simulink model "system_FIR_bank_decoder_AWGN"  (Simulink 8.3)
settings: Solver=ode45  StartTime=0.0  StopTime=10  RelTol=1e-3
undefined symbols (not defined in the file or in its folder): fdesignblkfcn, gcbh
libraries: commutil2 x2, commchan3 x1
(part 1 of 2)
settings Model: Creator=Vasilis  LastModifiedBy=Vasilis
settings OptimizationCC: ExpressionDepthLimit=2147483647
settings DebuggingCC: FcnCallInpInsideContextMsg=UseLocalSettings

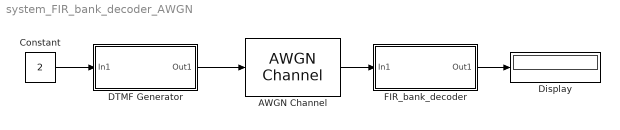
== system system_FIR_bank_decoder_AWGN ==
  AWGN Channel : commchan3/AWGN Channel  InputProcessing=Columns as channels (frame based)  seed=67  noiseMode="Signal to noise ratio  (SNR)"  EbNodB=10  EsNodB=10  SNRdB=-6  bitsPerSym=1  Ps=1  Tsym=1  variance=1
  Constant : Constant  Value=2
  DTMF Generator : Subsystem
  Display : Display
  FIR_bank_decoder : Subsystem
  wires:
  DTMF Generator/1(Out1) -> AWGN Channel/1
  FIR_bank_decoder/1(Out1) -> Display/1
  Constant/1 -> DTMF Generator/1(In1)
  AWGN Channel/1 -> FIR_bank_decoder/1(In1)

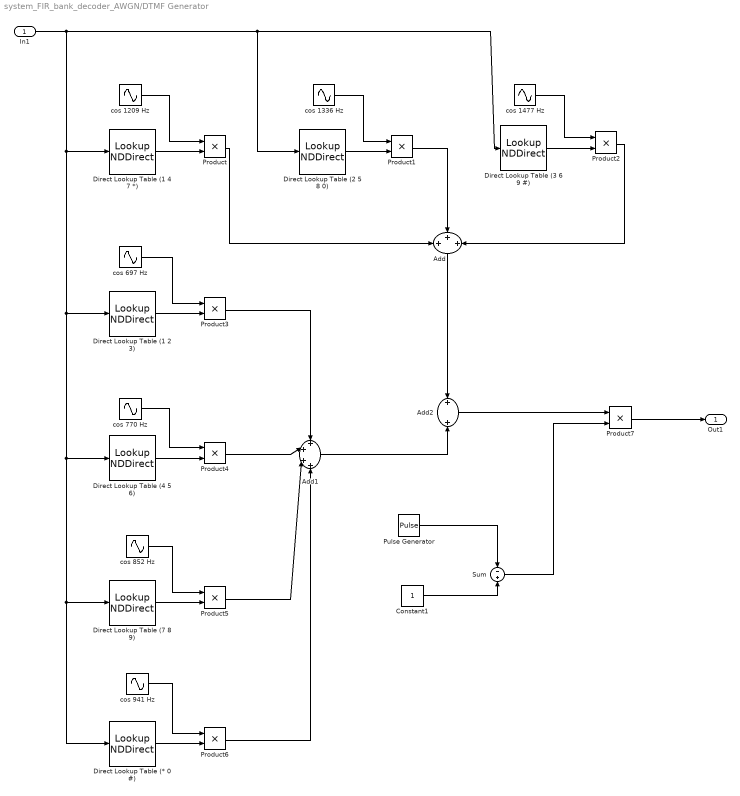
== system system_FIR_bank_decoder_AWGN/DTMF Generator ==
  In1 : Inport
  Add : Sum  Inputs=+++
  Add1 : Sum  Inputs=++++
  Add2 : Sum
  Constant1 : Constant
  Direct Lookup Table (* 0 #) : LookupNDDirect  NumberOfTableDimensions=1  Table=[1 0 0 0 0 0 0 0 0 0 1 1]
  Direct Lookup Table (1 2 3) : LookupNDDirect  NumberOfTableDimensions=1  Table=[0 1 1 1 0 0 0 0 0 0 0 0]
  Direct Lookup Table (1 4 7 *) : LookupNDDirect  NumberOfTableDimensions=1  Table=[0 1 0 0 1 0 0 1 0 0 1 0]
  Direct Lookup Table (2 5 8 0) : LookupNDDirect  NumberOfTableDimensions=1  Table=[1 0 1 0 0 1 0 0 1 0 0 0]
  Direct Lookup Table (3 6 9 #) : LookupNDDirect  NumberOfTableDimensions=1  Table=[0 0 0 1 0 0 1 0 0 1 0 1]
  Direct Lookup Table (4 5 6) : LookupNDDirect  NumberOfTableDimensions=1  Table=[0 0 0 0 1 1 1 0 0 0 0 0]
  Direct Lookup Table (7 8 9) : LookupNDDirect  NumberOfTableDimensions=1  Table=[0 0 0 0 0 0 0 1 1 1 0 0]
  Product{,1..7} (8 alike) : Product  RndMeth=Zero
  Pulse Generator : DiscretePulseGenerator  Period=480  PulseWidth=160  PhaseDelay=320  SampleTime=1/8000
  Sum : Sum  Inputs=-|+
  cos 1209 Hz : Sin  Frequency=7596  Phase=pi/2  SampleTime=1/8000
  cos 1336 Hz : Sin  Frequency=8394  Phase=pi/2  SampleTime=1/8000
  cos 1477 Hz : Sin  Frequency=9280  Phase=pi/2  SampleTime=1/8000
  cos 697 Hz : Sin  Frequency=4379  Phase=pi/2  SampleTime=1/8000
  cos 770 Hz : Sin  Frequency=4838  Phase=pi/2  SampleTime=1/8000
  cos 852 Hz : Sin  Frequency=5353  Phase=pi/2  SampleTime=1/8000
  cos 941 Hz : Sin  Frequency=5912  Phase=pi/2  SampleTime=1/8000
  Out1 : Outport
  wires:
  Direct Lookup Table (1 4 7 *)/1 -> Product/2
  In1/1 -> Direct Lookup Table (2 5 8 0)/1, Direct Lookup Table (3 6 9 #)/1, Direct Lookup Table (1 4 7 *)/1, Direct Lookup Table (1 2 3)/1, Direct Lookup Table (4 5 6)/1, Direct Lookup Table (7 8 9)/1, Direct Lookup Table (* 0 #)/1
  cos 1336 Hz/1 -> Product1/1
  Direct Lookup Table (2 5 8 0)/1 -> Product1/2
  cos 1477 Hz/1 -> Product2/1
  Direct Lookup Table (3 6 9 #)/1 -> Product2/2
  cos 697 Hz/1 -> Product3/1
  Direct Lookup Table (1 2 3)/1 -> Product3/2
  cos 770 Hz/1 -> Product4/1
  Direct Lookup Table (4 5 6)/1 -> Product4/2
  cos 852 Hz/1 -> Product5/1
  Direct Lookup Table (7 8 9)/1 -> Product5/2
  Product2/1 -> Add/3
  Product1/1 -> Add/2
  Product/1 -> Add/1
  Product3/1 -> Add1/1
  Product5/1 -> Add1/3
  Product4/1 -> Add1/2
  Add1/1 -> Add2/2
  Add/1 -> Add2/1
  cos 941 Hz/1 -> Product6/1
  Direct Lookup Table (* 0 #)/1 -> Product6/2
  Product6/1 -> Add1/4
  cos 1209 Hz/1 -> Product/1
  Constant1/1 -> Sum/2
  Pulse Generator/1 -> Sum/1
  Product7/1 -> Out1/1
  Add2/1 -> Product7/1
  Sum/1 -> Product7/2

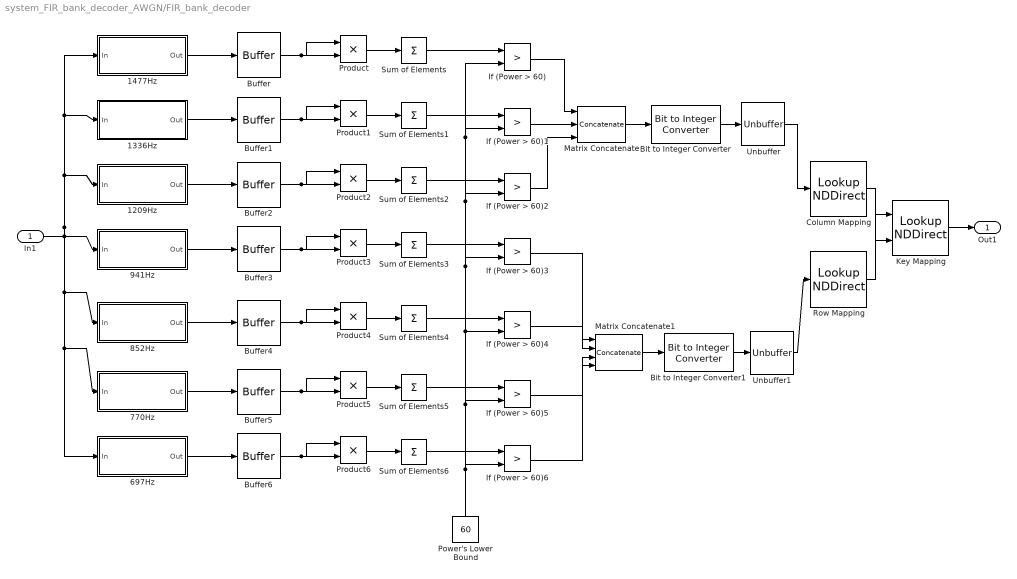
== system system_FIR_bank_decoder_AWGN/FIR_bank_decoder ==
  In1 : Inport
  1209Hz : Subsystem  DialogController=fdesignblkfcn  DialogControllerArgs=DataTag2  InitFcn=fdesignblkfcn(gcbh, {'InitFcn'});  mask(Bandpass Filter){}
      mask help: Design a bandpass filter
      settings: CopyFcn=fdesignblkfcn(gcbh, {'CopyFcn'});
      mask Help: helpview(mapfilelocation('dsp'), 'dspbandpassfilter');
      mask Display: disp('Bandpass');
  1336Hz : Subsystem  DialogController=fdesignblkfcn  DialogControllerArgs=DataTag4  InitFcn=fdesignblkfcn(gcbh, {'InitFcn'});  mask(Bandpass Filter){}
      mask help: Design a bandpass filter
      settings: CopyFcn=fdesignblkfcn(gcbh, {'CopyFcn'});
      mask Help: helpview(mapfilelocation('dsp'), 'dspbandpassfilter');
      mask Display: disp('Bandpass');
  1477Hz : Subsystem  DialogController=fdesignblkfcn  DialogControllerArgs=DataTag6  InitFcn=fdesignblkfcn(gcbh, {'InitFcn'});  mask(Bandpass Filter){}
      mask help: Design a bandpass filter
      settings: CopyFcn=fdesignblkfcn(gcbh, {'CopyFcn'});
      mask Help: helpview(mapfilelocation('dsp'), 'dspbandpassfilter');
      mask Display: disp('Bandpass');
  697Hz : Subsystem  DialogController=fdesignblkfcn  DialogControllerArgs=DataTag8  InitFcn=fdesignblkfcn(gcbh, {'InitFcn'});  mask(Bandpass Filter){}
      mask help: Design a bandpass filter
      settings: CopyFcn=fdesignblkfcn(gcbh, {'CopyFcn'});
      mask Help: helpview(mapfilelocation('dsp'), 'dspbandpassfilter');
      mask Display: disp('Bandpass');
  770Hz : Subsystem  DialogController=fdesignblkfcn  DialogControllerArgs=DataTag10  InitFcn=fdesignblkfcn(gcbh, {'InitFcn'});  mask(Bandpass Filter){}
      mask help: Design a bandpass filter
      settings: CopyFcn=fdesignblkfcn(gcbh, {'CopyFcn'});
      mask Help: helpview(mapfilelocation('dsp'), 'dspbandpassfilter');
      mask Display: disp('Bandpass');
  852Hz : Subsystem  DialogController=fdesignblkfcn  DialogControllerArgs=DataTag12  InitFcn=fdesignblkfcn(gcbh, {'InitFcn'});  mask(Bandpass Filter){}
      mask help: Design a bandpass filter
      settings: CopyFcn=fdesignblkfcn(gcbh, {'CopyFcn'});
      mask Help: helpview(mapfilelocation('dsp'), 'dspbandpassfilter');
      mask Display: disp('Bandpass');
  941Hz : Subsystem  DialogController=fdesignblkfcn  DialogControllerArgs=DataTag14  InitFcn=fdesignblkfcn(gcbh, {'InitFcn'});  mask(Bandpass Filter){}
      mask help: Design a bandpass filter
      settings: CopyFcn=fdesignblkfcn(gcbh, {'CopyFcn'});
      mask Help: helpview(mapfilelocation('dsp'), 'dspbandpassfilter');
      mask Display: disp('Bandpass');
  Bit to Integer Converter : commutil2/Bit to Integer Converter  nbits=3  bitOrder=MSB first  signedOutputValues=Unsigned  outDtype=Inherit via internal rule  outDtypeSigned=Inherit via internal rule
  Bit to Integer Converter1 : commutil2/Bit to Integer Converter  nbits=4  bitOrder=MSB first  signedOutputValues=Unsigned  outDtype=Inherit via internal rule  outDtypeSigned=Inherit via internal rule
  Buffer{,1..6} (7 alike) : Buffer  N=480  TreatMby1Signals=One channel
  Column Mapping : LookupNDDirect  NumberOfTableDimensions=1  Table=[0 1 2 0 3 0 0 0]
  If (Power > 60){,1..6} (7 alike) : RelationalOperator  Operator=>  OutDataTypeStr=boolean
  Key Mapping : LookupNDDirect  Table=[-1 -1 -1 -1;-1 1 2 3;-1 4 5 6;-1 7 8 9 ;-1 10 0 11]
  Matrix Concatenate : Concatenate  NumInputs=3  Mode=Multidimensional array
  Matrix Concatenate1 : Concatenate  NumInputs=4  Mode=Multidimensional array
  Power's Lower Bound : Constant  Value=60
  Product{,1..6} (7 alike) : Product  RndMeth=Zero
  Row Mapping : LookupNDDirect  NumberOfTableDimensions=1  Table=[0 1 2 0 3 0 0 4]
  Sum of Elements{,1..6} (7 alike) : Sum  Inputs=+
  Unbuffer : Unbuffer  SampleBasedProcessing=Same as frame based
  Unbuffer1 : Unbuffer  SampleBasedProcessing=Same as frame based
  Out1 : Outport
  wires:
  Product/1 -> Sum of Elements/1
  Buffer/1 -> Product/1, Product/2
  In1/1 -> 941Hz/1(In), 1477Hz/1(In), 1336Hz/1(In), 1209Hz/1(In), 852Hz/1(In), 697Hz/1(In), 770Hz/1(In)
  Product1/1 -> Sum of Elements1/1
  Buffer1/1 -> Product1/1, Product1/2
  Product2/1 -> Sum of Elements2/1
  Buffer2/1 -> Product2/1, Product2/2
  Buffer3/1 -> Product3/1, Product3/2
  Product4/1 -> Sum of Elements4/1
  Buffer4/1 -> Product4/1, Product4/2
  Product5/1 -> Sum of Elements5/1
  Buffer5/1 -> Product5/1, Product5/2
  Product6/1 -> Sum of Elements6/1
  Buffer6/1 -> Product6/1, Product6/2
  1477Hz/1(Out) -> Buffer/1
  1336Hz/1(Out) -> Buffer1/1
  1209Hz/1(Out) -> Buffer2/1
  941Hz/1(Out) -> Buffer3/1
  852Hz/1(Out) -> Buffer4/1
  770Hz/1(Out) -> Buffer5/1
  697Hz/1(Out) -> Buffer6/1
  Sum of Elements/1 -> If (Power > 60)/1
  Sum of Elements1/1 -> If (Power > 60)1/1
  Sum of Elements2/1 -> If (Power > 60)2/1
  Sum of Elements4/1 -> If (Power > 60)4/1
  Sum of Elements5/1 -> If (Power > 60)5/1
  Sum of Elements6/1 -> If (Power > 60)6/1
  Power's Lower Bound/1 -> If (Power > 60)6/2, If (Power > 60)5/2, If (Power > 60)4/2, If (Power > 60)3/2, If (Power > 60)2/2, If (Power > 60)1/2, If (Power > 60)/2
  If (Power > 60)/1 -> Matrix Concatenate/1
  If (Power > 60)1/1 -> Matrix Concatenate/2
  If (Power > 60)2/1 -> Matrix Concatenate/3
  If (Power > 60)4/1 -> Matrix Concatenate1/2
  If (Power > 60)5/1 -> Matrix Concatenate1/3
  If (Power > 60)6/1 -> Matrix Concatenate1/4
  Matrix Concatenate/1 -> Bit to Integer Converter/1
  Matrix Concatenate1/1 -> Bit to Integer Converter1/1
  Product3/1 -> Sum of Elements3/1
  Sum of Elements3/1 -> If (Power > 60)3/1
  If (Power > 60)3/1 -> Matrix Concatenate1/1
  Bit to Integer Converter/1 -> Unbuffer/1
  Bit to Integer Converter1/1 -> Unbuffer1/1
  Unbuffer1/1 -> Row Mapping/1
  Unbuffer/1 -> Column Mapping/1
  Column Mapping/1 -> Key Mapping/2
  Row Mapping/1 -> Key Mapping/1
  Key Mapping/1 -> Out1/1

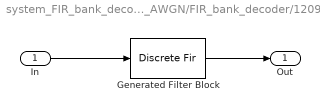
== system system_FIR_bank_decoder_AWGN/FIR_bank_decoder/1209Hz ==
  In : Inport
  Generated Filter Block : DiscreteFir  Tag=BlockMethodSubSystem  FilterStructure=Direct form symmetric  Coefficients=[0.0099903484009131061 -0.037287316277533809 -0.0082135057503011349 -0.002238399343519448 -0.0019360718453861063 -0.0019139958837784364 -0.00077884065160320319 0.00086714039520229187 0.0017467533892263094 0.0011565781392842288 -0.00039331281770252114 -0.0016111217199429831 -0.0014806300728323516 -0.00011463046784341615 0.0013522430913854087 0.0016917459634401887 0.0006177941951207149 -0.00098420252817349994 -0.0017744776461857054 -0.0010851913862388212 0.00052947391915747694 0.0017197450920395565 0.0014839755275524262 -1.0031615853397182e-05 -0.0015219092877656922 -0.001782126926066756 -0.0005405792693885126 0.0011845863495108277 0.0019528115419528134 0.0010844086186824026 -0.00072243441198573447 -0.0019705118995622111 -0.0015800809635293652 0.00015870918774939723 0.0018175461989234022 0.0019826643128734202 0.00047288121933751546 -0.0014893239615353924 -0.0022457206204821254 -0.0011229027958760288 0.00099697091022270408 0.0023348624407000793 0.0017391528527568611 -0.00036135984772205982 -0.0022193697097531986 -0.0022626461573520525 -0.00037321906555302491 0.0018887336645213278 0.002635976139918061 0.0011501753699652503 -0.0013470387071159013 -0.0028052485110882375 -0.0019156598422419128 0.00064021616557230205 0.0027033782721905563 0.0026066846174867754 0.00021123716890259276 -0.0023974935659959898 -0.0030588839233450706 -0.0011650031227231007 0.0017876927952893507 0.0033502764862502897 0.0020936796357518351 -0.00098985416249115408 -0.0033272963835514675 -0.0029002322095656764 -9.0731811744841788e-06 0.0029817669574168006 0.0035380445077329505 0.0011180900776899118 -0.0023355724129337395 -0.0039190793929641419 -0.00222802286610753 0.001416890805220176 0.0039702899594947919 0.0032339842000296986 -0.00027747486969317007 -0.0036560247606840408 -0.0040323809948562255 -0.00099397563382286162 0.0029719075272680536 0.0045309986988746357 0.0022857605388528395 -0.001957886965572142 -0.0046645685103582678 -0.0034878823319817332 0.00067864161875333753 0.0043947083433336894 0.0044975321496961889 0.0008070250875256077 -0.0036547196147583149 -0.0051275760337421167 -0.0022940033180403599 0.0025597990824570661 0.0053678498199717832 0.0037063460007083961 -0.0011371111116267032 -0.0051335228642123429 -0.0048859611206101888 -0.00049200244291961739 0.0044169937498863008 0.0057120234201003704 0.0021964902927675964 -0.0032476121239446453 -0.0060817475478434696 -0.0038258197948308576 0.0017078844412512415 0.0059189980367584218 0.005226507870014001 8.9398956346120948e-05 -0.0052181801450817368 -0.006234351203697289 -0.0020091131071094991 0.0040058848539415211 0.00675549284565982 0.0038506474059017038 -0.0023528353020247964 -0.0066897155494656671 -0.0054674949837762183 0.0003934727850060219 0.0060319185594673247 0.0066788774561016692 0.0017030867964629001 -0.0047911800779544544 -0.0073570236405915666 -0.0037665296571841715 0.0030569414532184568 0.0074177453956615746 0.0055994350622296648 -0.00096978489582727988 -0.0068249732831169125 -0.0070175194579185579 -0.0013021135874790543 0.0055941410556593092 0.0078790462315889952 0.0035628144520170814 -0.0038102632589340174 -0.0080797022380677055 -0.0056059555558007589 0.0016183821021101376 0.0075780000877349292 0.007241559943165804 0.00080784635882471081 -0.0063844597921917387 -0.0082962272924075684 -0.0032512084061216287 0.0045864365088574425 0.0086572921505485706 0.0054936294742238068 -0.002322420975806325 -0.008271267955622965 -0.0073321411791402603 -0.000222805070376603 0.0071457333019116212 0.008586878232170558 0.0028257738862537958 -0.0053600683209759758 -0.0091258191828687413 -0.0052565101689838432 0.0030554117960418666 0.0088770115844641912 0.0072973186248119857 -0.00042562852809473011 -0.0078493123308107163 -0.0087475340501937966 -0.0023104884567685291 0.0061148064953200562 0.0094682866573189001 0.0049040210729837551 -0.0038007366415396086 -0.0093788089591992294 -0.0071250481351540617 0.0011174650996554102 0.0084669741911153461 0.008755897555957565 0.0017074331947345644 -0.0068136230101083382 ...(+5049 chars)]  InputProcessing=Columns as channels (frame based)
  Out : Outport
  wires:
  In/1 -> Generated Filter Block/1
  Generated Filter Block/1 -> Out/1

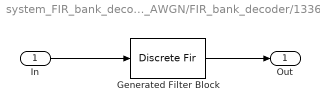
== system system_FIR_bank_decoder_AWGN/FIR_bank_decoder/1336Hz ==
  In : Inport
  Generated Filter Block : DiscreteFir  Tag=BlockMethodSubSystem  FilterStructure=Direct form symmetric  Coefficients=[0.027095683988763684 -0.02145962611614876 -0.013237259442949369 -0.0087875280000578541 -0.0072025518691899455 -0.0064053551512149535 -0.0046877492747228709 -0.0020678117191547346 1.5783089193229684e-05 0.00029058250509216379 -0.0009461225532965765 -0.002076158370976302 -0.0016998189397077492 -1.7135878450373401e-05 0.0014180811397398326 0.0012425739522998588 -0.00031259540690893486 -0.0016611531037952992 -0.0014072875825471226 0.00022516620337938411 0.0016295385369482407 0.001384181168339018 -0.00027617786866151718 -0.001702408224554393 -0.001433466449239222 0.00028636498762473048 0.0017588912746925752 0.0014735010392152908 -0.00031181837932445119 -0.0018360050467830125 -0.0015270612311243344 0.00033502107081047583 0.001920012269702764 0.0015843826985173222 -0.0003629922298134779 -0.0020196099323054814 -0.0016468399430713846 0.00038494436810798438 0.0021318241990705864 0.0017204393872174025 -0.00044364818722663295 -0.0022038343728180863 -0.0018389996862307749 0.0004747245180321579 0.0023649199696544531 0.0018956816680701684 -0.00053084319789423011 -0.0024775400450006437 -0.0019789719623437771 0.00055672915937643528 0.0026099326449985538 0.0020833438006598454 -0.00059848464364556321 -0.0027655971720919326 -0.0021895280734174948 0.00065250840029930531 0.002925473812108891 0.0022912874900265123 -0.00071125565894482789 -0.0030861784329826616 -0.0023912894204413618 0.00077374918196846114 0.0032516700984419268 0.002495791726490506 -0.00083470618733626884 -0.0034202484186360632 -0.0026037101295327391 0.00089877837036419475 0.0035974309999007338 0.0027175235283487774 -0.00096345645417326661 -0.0037779122225057777 -0.0028341889227190041 0.0010283895960031448 0.0039608531736712834 0.0029513791481683965 -0.0011002355614192524 -0.0041438537084830824 -0.003073356575340881 0.0011772022921241604 0.0043305752920002006 0.0031750438811959541 -0.0012522821857654228 -0.0045366334501035482 -0.0032884278657823759 0.0013520119224747452 0.0047405753007125333 0.0034032910697775862 -0.001433739052490146 -0.0049482205885360902 -0.0035309378393161431 0.0015177933231502426 0.0051548972798418696 0.0036460961897361202 -0.0016073700516777744 -0.0053503669589460663 -0.0037464114490644621 0.0017063964907911343 0.0055551413794671066 0.0038555149718838824 -0.0018045808744347671 -0.0057668678811651636 -0.0039722023906121947 0.0018956865971788426 0.0059685707953339448 0.0040773353033411374 -0.0019941908115179486 -0.0061686032214466249 -0.0041728971415513532 0.0021037574851192533 0.0063746362282919135 0.0042720026838175872 -0.0022084554659246121 -0.0065767872093308909 -0.0043731862282702519 0.002307693019411501 0.0067689507813790137 0.0044588442550910603 -0.0024137927254855129 -0.0069690457781116542 -0.0045423086107703927 0.0025256799060105603 0.0071664825013771317 0.0046374216101847041 -0.0026300818482279916 -0.0073550948665105833 -0.0047127819534048985 0.0027389156670564936 0.0075383476067156984 0.0047881089571674218 -0.0028545987991045766 -0.007730395950912794 -0.004864088876636496 0.0029645336738986692 0.0079070996628302099 0.0049287940432560023 -0.0030727103204409765 -0.0080771259141469744 -0.0049876532964567635 0.0031876311620945069 0.0082527679043450219 0.0050492371353173067 -0.0032958435304926903 -0.0084131178482600884 -0.005096428485431093 0.0034077038789324956 0.0085693134242927141 0.0051398427379930074 -0.0035203051186928152 -0.0087255003594660582 -0.0051867130753659616 0.0036211036523363374 0.0088646141369722511 0.0052190498440896063 -0.0037289944365722842 -0.0090066415144954663 -0.0052492206781625424 0.003833583157621718 0.0091363028340680219 0.00527569360828013 -0.0039353903470793622 -0.0092517108051435124 -0.0052858981004161153 0.0040430002734167716 0.0093750585558239237 0.0053055527387765346 -0.0041374757743999173 -0.0094745654534143103 -0.0053071456503114038 0.0042376341409502511 0.0095793767923593575 0.0053118055532269046 -0.0043305699638566128 -0.0096691116603148438 -0.0053081962230121351 0.0044152806449220374 0.009742329148113996 ...(+5036 chars)]  InputProcessing=Columns as channels (frame based)
  Out : Outport
  wires:
  In/1 -> Generated Filter Block/1
  Generated Filter Block/1 -> Out/1

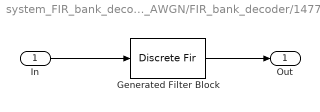
== system system_FIR_bank_decoder_AWGN/FIR_bank_decoder/1477Hz ==
  In : Inport
  Generated Filter Block : DiscreteFir  Tag=BlockMethodSubSystem  FilterStructure=Direct form symmetric  Coefficients=[-0.0287532521465266 0.018950539278399056 0.01226030961531808 0.0089462510732899424 0.0080720399029321332 0.0071063372274715883 0.0046332180233575257 0.0017273609418207039 0.00049665842142506246 0.0013871322506781513 0.0025979362385936092 0.0021324146084545021 0.00016669053741646259 -0.0012372978388415965 -0.00058929149978922263 0.0011803290377975025 0.0018482274584829814 0.00050653851927123838 -0.0012982717331836843 -0.0014450254947155844 0.0002460064873962881 0.0017266496604581257 0.0011930072485507725 -0.00077012760084695618 -0.0018095795084877044 -0.0006623403084351576 0.0013383536401150526 0.0017645537338465008 6.9190011544951999e-05 -0.0017586939105366057 -0.0014830587794361345 0.00060220048023955884 0.002028130564433372 0.0010142052415943368 -0.0012537074198326614 -0.0020805631301777203 -0.00037526045156384869 0.0018301068017267663 0.0018699113285282909 -0.00033694206578713872 -0.0022745680256688102 -0.0014345621319109478 0.0011594598093304879 0.002417914479003557 0.00077387705731969453 -0.0018646259010602214 -0.002333943763047804 3.3362549135409694e-05 0.0024495735101620823 0.0019598695598750269 -0.00095296170141684355 -0.0028060011624454519 -0.0012901762655438511 0.0018600551822057548 0.0028450720937096773 0.00038300047356122077 -0.0026322754682392082 -0.0025335878798225862 0.0006643306307372918 0.0031595414553335314 0.001880945893506004 -0.0017368124624291884 -0.0033532190403897382 -0.00093063780129923714 0.0027090098772565574 0.0031573349878150775 -0.00023296024663496277 -0.0034508512401011048 -0.0025544092961549197 0.0014911494434784508 0.003853063008719391 0.0015809136309946055 -0.002693847458814823 -0.0038295536005158136 -0.0003204835852551771 0.0036826959037909676 0.0033306911867856527 -0.0010903280438726243 -0.0043199459334335851 -0.0023657086442658067 0.0025131226259623406 0.0044730484449647572 0.0010357162674199487 -0.0037682874440775828 -0.0041170820080304949 0.00054972751233127166 0.0046796444258475544 0.0032264188138248812 -0.0021892992948818048 -0.0050792467871731539 -0.0018647081156969324 0.0036993409513402069 0.0049023859520455444 0.00016530942934150165 -0.0048968835012872958 -0.0041305491231340401 0.0016823513552986955 0.0055952518292413603 0.0028008223656188712 -0.0034619692212331356 -0.0056590272879834093 -0.001025698986503505 0.0049604171151156019 0.0050507983876609966 -0.00099544716148336249 -0.0059709843855467052 -0.0038056520910975302 0.0030238973558277113 0.0063275917210827599 0.0020173029746219612 -0.0048266583643151624 -0.0059526939548204764 0.00013235573819970993 0.0061777059444965733 0.0048580288472332509 -0.0023841047346674429 -0.0068713872699185524 -0.0031093835699988232 0.0044872068945739779 0.0067830034820160756 0.00089035024956171725 -0.0061939627549512169 -0.0058971503858197237 0.0015492106439668652 0.0072445273836480514 0.0042609204425713499 -0.0039299924920481481 -0.007492755528533299 -0.0020345578492505316 0.0059790620880847889 0.0068821120338397454 -0.00053264574435280963 -0.0074102017919554361 -0.0054202628215857442 0.0031586579722530884 0.0080351121822384314 0.0032552145116494006 -0.0055336868430688416 -0.0077555144415542608 -0.0006316645228711511 0.0073481362134504838 0.0065445180348209534 -0.0021840010035608232 -0.0083845299655538365 -0.0045260112634828665 0.0048493458383536232 0.0084764752289131357 0.0019046657632195096 -0.0070378094665666524 -0.0075748443211424727 0.0010377648004505566 0.0084871130827781447 0.0057691197245270777 -0.0039501476627919344 -0.008996959108926967 -0.0032381246038995061 0.0064794660700983617 0.0084625251873871477 0.00024390476700450434 -0.0083481571802224916 -0.0069449410101073035 0.0028427735509807235 0.0092774086142669056 0.0045659962091380421 -0.0056947290932644621 -0.009170813710900335 -0.0016153705337077877 0.007938890259920903 0.0079864282280410603 -0.001594140752776047 -0.009312113264207748 -0.0058585005424023756 0.0046772554323861251 0.0096360810037030876 0.0030121914666760537 -0.0072795786239457979 -0.0088582260427276273 ...(+5034 chars)]  InputProcessing=Columns as channels (frame based)
  Out : Outport
  wires:
  In/1 -> Generated Filter Block/1
  Generated Filter Block/1 -> Out/1

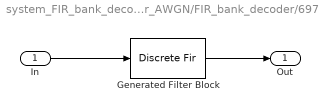
== system system_FIR_bank_decoder_AWGN/FIR_bank_decoder/697Hz ==
  In : Inport
  Generated Filter Block : DiscreteFir  Tag=BlockMethodSubSystem  Coefficients=[0.012186060064151707 -0.055647365743080338 -0.011622923542949751 -0.0023601443159607443 -0.00037709321297497549 5.3192570035937454e-05 9.5306644539136783e-05 -4.3886654722388434e-07 -0.00016698516531360265 -0.00033240566929396761 -0.0004339367718662525 -0.00040936875260382644 -0.000242891174569655 4.3305826211138289e-05 0.00036633163701552818 0.00063114458575970402 0.00073024435767673817 0.00061593525776928516 0.00028778759346346393 -0.00017100912517735388 -0.00063557207014733818 -0.00095238933880689551 -0.0010112426735624652 -0.00075791145635616098 -0.00025033233027123422 0.00038836279593825363 0.00096030981013857342 0.0012922885731270776 0.0012520241177654393 0.00082896229662711874 0.00011680727272044896 -0.00068097210032956254 -0.0013331378114595407 -0.0016216153004023862 -0.0014429140840378648 -0.00080889613042098134 0.00010466310433670427 0.0010496763521975676 0.001729572012124053 0.0019337793004115941 0.0015607749894947002 0.0007025980137055981 -0.0004217489004241364 -0.0014714469110599963 -0.0021447009101689131 -0.0021977329863294816 -0.0016043873363791145 -0.0004879461700825842 0.0008149518360261299 0.0019537992627646442 0.0025383747647199483 0.0024222667387726227 0.0015264942756827555 0.0002075367187239933 -0.0013273975579545835 -0.0024276376043035363 -0.0029213489278016799 -0.0025686294285510967 -0.0013523648399656047 0.00021999826598754045 0.0018163564571418494 0.0029736583028155978 0.003275902544143657 0.0025676851481386321 0.0010994918991200568 -0.00072698715758976276 -0.0024052920366846925 -0.0034643932751787774 -0.0035294315996001052 -0.0025395642321969342 -0.00073982324218347544 0.001336011079998791 0.0030783291454537618 0.003951430072754311 0.0036834139503892751 0.002312751434488408 0.00022513929617226655 -0.0019976278408449259 -0.0036912200454956509 -0.0043491092797696366 -0.0037348764983612024 -0.0019975709249641324 0.00038645239460916568 0.0027265390450931766 0.0043334471113618718 0.0047065794477740737 0.0037067702527548737 0.0015834527657456444 -0.0010593958798154235 -0.0034622047740676524 -0.0049021032066739476 -0.0049357420479861332 -0.0035120100426779288 -0.0010194615112873724 0.00183966580642867 0.004222513194134153 0.0054232934968280952 0.0050503824248528083 0.003187010966381553 0.00033606528152412137 -0.0026751690671439707 -0.0049733965160602732 -0.0058531972422194746 -0.005041193654796835 -0.0027174594559769985 0.00044257350272483445 0.0035562984580145857 0.0056761364591739723 0.0061834823388317584 0.0048874019008518788 0.0021136999654420095 -0.0013106488143002624 -0.0044456673713511603 -0.0063228355777168828 -0.0063807483004715464 -0.0045795660759258951 -0.0013964556565729046 0.0022647269208475682 0.0053159471956116533 0.0068680468155390842 0.0064424749962669762 0.0041225594762825954 0.0005450752303490711 -0.0032460011042601167 -0.0061452441133167989 -0.0073010636679993191 -0.0063470503537903797 -0.003514996881178253 0.00039234325409859191 0.0042490422484621751 0.0069141714126522598 0.0076002761482082837 0.0060801917918021477 0.0027633491755993602 -0.001408504431109109 -0.0052344450907843756 -0.0075851268858776839 -0.0077525999641170039 -0.0056566585399264319 -0.0018805632554488544 0.0024902849866272488 0.0061884036511721235 0.0081264468530882553 0.0077208619362845671 0.0050621038769007127 0.0008973260962082066 -0.0035795547288231737 -0.0070648616533375294 -0.0085326523043507459 -0.0075288831613373186 -0.0043240750073869081 0.00017464383745750473 0.0046688431301704688 0.0078519014111278658 0.0087797672999804562 0.0071630038467761789 0.0034452010171803064 -0.0013044689851883266 -0.0057210298737931098 -0.0085114479824384623 -0.0088496006002427054 -0.0066213214499983072 -0.0024447085055165426 0.0024625698092206878 0.0067051035067572104 0.0090197511798191157 0.0087330223733588837 0.0059101452475405509 0.0013465132186586634 -0.0036364350968752304 -0.0075949164341442433 -0.0093777473384244678 -0.0084453365175865269 -0.0050583145554218894 -0.00018575121084798933 0.0047676588026061258 ...(+5081 chars)]  InputProcessing=Columns as channels (frame based)
  Out : Outport
  wires:
  In/1 -> Generated Filter Block/1
  Generated Filter Block/1 -> Out/1
